simulink model "sia003A"  (R2023b)
settings: Solver=VariableStepAuto  StartTime=0.0  StopTime=10  FixedStep=0.001  RelTol=1e-3  EnableMultiTasking=on
values from neighbouring files (symbols this model uses):
  a1 = 0.040    (= 0.04)    [run_feedforward_experiment.m]
  a2 = 0.275    [run_feedforward_experiment.m]
  a3 = 0.025    [run_feedforward_experiment.m]
  d4 = 0.280    (= 0.28)    [run_feedforward_experiment.m]
  m = [0.167, 1, 0.5, 0.333, 0.25, 0.2]    [run_feedforward_experiment.m]
undefined symbols (not defined in the file or in its folder): d1, fc1, fc2, fc3, fc4, fc5, fc6, fv1, fv2, fv3, fv4, fv5, fv6, Ia1, Ia2, Ia3, Ia4, Ia5, Ia6, Ic111, Ic112, Ic113, Ic122, Ic123, Ic133, Ic211, Ic212, Ic213, Ic222, Ic223, Ic233, Ic311, Ic312, Ic313, Ic322, Ic323, Ic333, Ic411, Ic412, Ic413, Ic422, Ic423, Ic433, Ic511, Ic512, Ic513, Ic522, Ic523, Ic533, Ic611, Ic612, Ic613, Ic622, Ic623, Ic633, m1, m2, m3, m4, m5 ... (+22)
libraries: sm_lib x56, nesl_utility x31, slpidlib x12, simulink x8
(part 3 of 3)

== matlab function sia003A/Robot/Robot/robot/friction ==
  data: u input; y output; fv input; fc input
function y = fcn(u,fv,fc)
%#codegen


% fv1=100; fc1=80; fv2=150; fc2=100; fv3=100; fc3=50; fv4=80; fc4=80; fv5=50; fc5=30; fv6=30; fc6=10;
fv1=fv(1); fc1=fc(1); fv2=fv(2); fc2=fc(2); fv3=fv(3); fc3=fc(3); fv4=fv(4); fc4=fc(4); fv5=fv(5); fc5=fc(5); fv6=fv(6); fc6=fc(6);
y=[0;0;0;0;0;0];
y(1)=(fv1*u(1)+fc1*sign(u(1)));
y(2)=(fv2*u(2)+fc2*sign(u(2)));
y(3)=(fv3*u(3)+fc3*sign(u(3)));
y(4)=(fv4*u(4)+fc4*sign(u(4)));
y(5)=(fv5*u(5)+fc5*sign(u(5)));
y(6)=(fv6*u(6)+fc6*sign(u(6)));

end

== matlab function sia003A/Robot/Robot/robot/Jm ==
  data: u input; y output; Jm input
function y = fcn(u,Jm)
%#codegen

% Jm=[200; 250; 150; 100; 50; 20];%关节惯性
y = Jm.*u;
end

== matlab function sia003A/周期信号发生器 ==
  data: Amplitude parameter; Bias parameter; Frequency parameter; Phase parameter; out output; t_in input
function out=PeriodicSignallGenerator(Amplitude,Bias,Frequency, Phase,t_in)

    [m,n]=size(Amplitude);
    Amplitude=reshape(Amplitude,m*n,1);
    Bias=reshape(Bias,m*n,1);
    Frequency=reshape(Frequency,m*n,1);
    Phase=reshape(Phase,m*n,1);
    %规划
	ss=zeros(m*n,1);
	se=Amplitude;
	vs=zeros(m*n,1);
	ve=zeros(m*n,1);
	as=zeros(m*n,1);
	ae=zeros(m*n,1);
	js=zeros(m*n,1);
	je=zeros(m*n,1);
	tend=0.25./Frequency;

	tf=tend;
	tf2=tend.*tend;
	tf3=tend.*tend.*tend;
	tf4=tend.*tend.*tend.*tend;
	tf5=tend.*tend.*tend.*tend.*tend;
	tf6=tend.*tend.*tend.*tend.*tend.*tend;
	tf7=tend.*tend.*tend.*tend.*tend.*tend.*tend;

	b1=se-js./6.0.*tf3 - as./2.0.*tf2 - vs.*tf - ss;
	b2=ve-js./2.0.*tf2 - as.*tf - vs;
	b3=ae-js.*tf - as;
	b4=je-js;

    a=zeros(m*n,8);
	a(:,1)=ss;
	a(:,2)=vs;
	a(:,3)=as./2.0;
	a(:,4)=js./6.0;
	a(:,5)=(35.*b1)./tf4 - (15.*b2)./tf3 + (5.*b3)./(2.*tf2) - b4./(6.*tf);
	a(:,6)=(39.*b2)./tf4 - (84.*b1)./tf5 - (7.*b3)./tf3 + b4./(2.*tf2);
	a(:,7)=(70.*b1)./tf6 - (34.*b2)./tf5 + (13.*b3)./(2.*tf4) - b4./(2.*tf3);
	a(:,8)=(10.*b2)./tf6 - (20.*b1)./tf7 - (2.*b3)./tf5 + b4./(6.*tf4);
    
    %
    t_=zeros(m*n,1);
    t=zeros(m*n,1);
    ts=1.0./Frequency;
	t14=ts./4.0;
	t24=ts./2.0;
	t34=3.*ts./4.0;
	t44=ts;
	
    sign_=ones(m*n,1);
    %   
    for k=1:m*n
        t(k)=t_in+Phase(k);
        if (t(k)<0)
            sign_(k)=-1;
            t(k)=-t(k);
        end
        t(k)=t(k)-floor(t(k)/ts(k))*ts(k);
        if ((t(k)>=0)&&(t(k)<t14(k)))
            t_(k)=t(k);
        end
        if ((t(k)>=t14(k))&&(t(k)<t24(k)))
             t_(k)=t24(k)-t(k); 
        end
        if((t(k)>=t24(k))&&(t(k)<t34(k)))
             t_(k)=t(k)-t24(k);
             sign_(k)=-1.*sign_(k);
        end
        if((t(k)>=t34(k)))
             t_(k)=t44(k)-t(k);
             sign_(k)=-1.*sign_(k);        
        end
    

        if (t(k)>tend(k))
            t(k)=tend(k);
        end
        if (t(k)<0)
            t(k)=0;
        end
    end

    
	t2=t_.*t_;
	t3=t_.*t_.*t_;
	t4=t_.*t_.*t_.*t_;
	t5=t_.*t_.*t_.*t_.*t_;
	t6=t_.*t_.*t_.*t_.*t_.*t_;
	t7=t_.*t_.*t_.*t_.*t_.*t_.*t_;

	out =a(:,8).*t7 + a(:,7).*t6 + a(:,6).*t5 + a(:,5).*t4 + a(:,4).*t3 + a(:,3).*t2 + a(:,2).*t + a(:,1);
	out=sign_.*out+Bias;

end

== matlab function sia003A/dynamics + PID Control/Idynamics/Robot Dynamics ==
  data: q input; T output; qd input; qdd input

function T   = Idynamics( q,qd,qdd )
offset2=-pi/2;

s1=sin(q(1)); c1=cos(q(1)); 
s2=sin(q(2)+offset2); c2=cos(q(2)+offset2);
s3=sin(q(3)); c3=cos(q(3));
s4=sin(q(4)); c4=cos(q(4));
s5=sin(q(5)); c5=cos(q(5));
s6=sin(q(6)); c6=cos(q(6));

Q11=qd(1);  Q21=qd(2);  Q31=qd(3);  Q41=qd(4);  Q51=qd(5);  Q61=qd(6); 
Q12=qdd(1);  Q22=qdd(2);  Q32=qdd(3);  Q42=qdd(4);  Q52=qdd(5);  Q62=qdd(6);
f71=0;  f72=0;  f73=0;  n71=0;  n72=0;  n73=0;

%---------------------------------设置参数--------------------------------

% m1=0.00100000000000000;  m2=0.00100000000000000;  m3=0.00100000000000000;  m4=0.00100000000000000;  m5=0.00100000000000000;  m6=0.00100000000000000;
% 
% mc11=0;  mc12=0;  mc13=0;
% mc21=4651.50225394466;  mc22=-131.825587047461;  mc23=0;
% mc31=-60.5441532996453;  mc32=674.258060919694;  mc33=0;
% mc41=18.7559635838501;  mc42=-8.94631572009627;  mc43=0;
% mc51=39.1850949869383;  mc52=70.3651817994520;  mc53=0;
% mc61=-9.46764788612443;  mc62=-36.4261551831934;  mc63=0;%质心位置
% 
% 
% Ic111=0;  Ic122=0;  Ic133=2580.391811604250;  Ic112=0;  Ic113=0;  Ic123=0;
% Ic211=-2308.54980136788;  Ic222=-21636.4732184523;  Ic233=-19427.4931578430;  Ic212=-655.299381991673;  Ic213=-402.481626864736;  Ic223=1625.61432421119;
% Ic311=177.446872113322;  Ic322=-3.66559449877095;  Ic333=1225.66014585809;  Ic312=1065.32242628535;  Ic313=135.253022811379;  Ic323=-212.654795897439;
% Ic411=-856.449748636182;  Ic422=-0.351786169958710;  Ic433=637.546049655485;  Ic412=17.6321938869444;  Ic413=432.315615848409;  Ic423=528.159872075546;
% Ic511=53.5070403383571;  Ic522=-1.53547166913538;  Ic533=-275.931221064706;  Ic512=43.6352272669739;  Ic513=-110.142321946823;  Ic523=-292.481991287130;
% Ic611=89.4468595890859;  Ic622=-0.0896363564956364;  Ic633=183.333947383574;  Ic612=-31.1239742083191;  Ic613=40.1733539538204;  Ic623=-0.510715170309807;%惯性矩
% 
% g=9802.00;
% 
% %XB4
% % d1=342;a1=40;a2=275;a3=25;d4=280;dt=73;
% %XB6
% % d1=380;a1=30;a2=340;a3=35;d4=345;dt=90;
% %XB7
% d1=380;a1=30;a2=340;a3=35;d4=345;dt=87;
% 
% Ia1=0; Ia2=0; Ia3=-381.979781193985; Ia4=-848.046494253400; Ia5=106.880560008008; Ia6=-553.016107704353;%关节惯性
% fv1=14300.3219938765; fc1=10364.8985579369; fv2=77554.0985985479; fc2=17597.4704449446; fv3=13127.7878719491; fc3=8947.89951285878; 
% fv4=3252.91588327327; fc4=4394.56545040839; fv5=5533.12349479137; fc5=2614.97320533832; fv6=2209.46946763177; fc6=4156.29047300509;%粘滞摩擦,库伦摩擦

% m1=1.00000000000000;  m2=1.00000000000000;  m3=1.00000000000000;  m4=1.00000000000000;  m5=1.00000000000000;  m6=1.00000000000000;
% 
% mc11=0;  mc12=0;  mc13=0;
% mc21=4.65150225394466;  mc22=-0.131825587047461;  mc23=0;
% mc31=-0.0605441532996453;  mc32=0.674258060919694;  mc33=0;
% mc41=0.0187559635838501;  mc42=-0.00894631572009627;  mc43=0;
% mc51=0.0391850949869383;  mc52=0.0703651817994520;  mc53=0;
% mc61=-0.00946764788612443;  mc62=-0.0364261551831934;  mc63=0;%质心位置
% 
% Ic111=0;  Ic122=0;  Ic133=2.580391811604250;  Ic112=0;  Ic113=0;  Ic123=0;
% Ic211=-2.30854980136788;  Ic222=-21.6364732184523;  Ic233=-19.4274931578430;  Ic212=-0.655299381991673;  Ic213=-0.402481626864736;  Ic223=1.62561432421119;
% Ic311=0.177446872113322;  Ic322=-0.00366559449877095;  Ic333=1.22566014585809;  Ic312=1.06532242628535;  Ic313=0.135253022811379;  Ic323=-0.212654795897439;
% Ic411=-0.856449748636182;  Ic422=-0.000351786169958710;  Ic433=0.637546049655485;  Ic412=0.0176321938869444;  Ic413=0.432315615848409;  Ic423=0.528159872075546;
% Ic511=0.0535070403383571;  Ic522=-0.00153547166913538;  Ic533=-0.275931221064706;  Ic512=0.0436352272669739;  Ic513=-0.110142321946823;  Ic523=-0.292481991287130;
% Ic611=0.0894468595890859;  Ic622=-0.0000896363564956364;  Ic633=0.183333947383574;  Ic612=-0.0311239742083191;  Ic613=0.0401733539538204;  Ic623=-0.000510715170309807;%惯性矩
% 
% g=9.80200;
% 
% %XB4
% % d1=342;a1=40;a2=275;a3=25;d4=280;dt=73;
% %XB6
% % d1=380;a1=30;a2=340;a3=35;d4=345;dt=90;
% %XB7
% d1=0.380;a1=0.030;a2=0.340;a3=0.035;d4=0.345;dt=0.087;
% 
% Ia1=0; Ia2=0; Ia3=-0.381979781193985; Ia4=-0.848046494253400; Ia5=0.106880560008008; Ia6=-0.553016107704353;%关节惯性
% fv1=14.3003219938765; fc1=10.3648985579369; fv2=77.5540985985479; fc2=17.5974704449446; fv3=13.1277878719491; fc3=8.94789951285878; 
% fv4=3.25291588327327; fc4=4.39456545040839; fv5=5.53312349479137; fc5=2.61497320533832; fv6=2.20946946763177; fc6=4.15629047300509;%粘滞摩擦,库伦摩擦
% 
% % Ia1=0; Ia2=0; Ia3=0; Ia4=0; Ia5=0; Ia6=0;%关节惯性
% % fv1=0; fc1=0; fv2=0; fc2=0; fv3=0; fc3=0; 
% % fv4=0; fc4=0; fv5=0; fc5=0; fv6=0; fc6=0;%粘滞摩擦,库伦摩擦

m1=0.167;  m2=1;  m3=0.5;  m4=0.333;  m5=0.25;  m6=0.2;

mc11=0;  mc12=0;  mc13=0.2;
mc21=0.1291;  mc22=0;  mc23=3.3117;
mc31=1.6484;  mc32=0;  mc33=0.8748;
mc41=0.3200;  mc42=0.2324;  mc43=0.7083;
mc51=0.4574;  mc52=0;  mc53=0.6427;
mc61=0.3200;  mc62=-0.0513;  mc63=0.6417;%质心位置

Ic111=0;  Ic122=0;  Ic133=1.3676;  Ic112=0;  Ic113=0;  Ic123=0;
Ic211=8.8194;  Ic222=6.0549;  Ic233=0.9569;  Ic212=0;  Ic213=0;  Ic223=0;
Ic311=0.0332;  Ic322=1.8442;  Ic333=1.0560;  Ic312=0;  Ic313=0;  Ic323=0;
Ic411=0.1448;  Ic422=0.0015;  Ic433=0.0822;  Ic412=0;  Ic413=0;  Ic423=0;
Ic511=0;  Ic522=0.0121;  Ic533=0.0299;  Ic512=0;  Ic513=0;  Ic523=0;
Ic611=0.0134;  Ic622=0;  Ic633=0.0051;  Ic612=0;  Ic613=0;  Ic623=0;%惯性矩

g=9.80200;

%XB4
d1=0.342;a1=0.040;a2=0.275;a3=0.025;d4=0.280;dt=0.073;
%XB6
% d1=380;a1=30;a2=340;a3=35;d4=345;dt=90;
%XB7
% d1=0.380;a1=0.030;a2=0.340;a3=0.035;d4=0.345;dt=0.087;

Ia1=0; Ia2=0; Ia3=0; Ia4=0; Ia5=0; Ia6=0;%关节惯性
fv1=0; fc1=0; fv2=0; fc2=0; fv3=0; fc3=0; 
fv4=0; fc4=0; fv5=0; fc5=0; fv6=0; fc6=0;%粘滞摩擦,库伦摩擦



R01=[c1 -s1 0;
    s1 c1 0;
    0 0 1];
R12=[c2 -s2 0;
    0 0 1;
    -s2 -c2 0];
R23=[c3 -s3 0;
    s3 c3 0;
    0 0 1];
R34=[c4 -s4 0;
    0 0 1;
    -s4 -c4 0];
R45=[c5 -s5 0;
    0 0 -1;
    s5 c5 0];
R56=[c6 -s6 0;
    0 0 1;
    -s6 -c6 0];
R06=R01*R12*R23*R34*R45*R56;
R10=R01';R21=R12';R32=R23';R43=R34';R54=R45';R65=R56';
%R67=eye(3);

QZ1=[0;0;Q11];QZ2=[0;0;Q21];QZ3=[0;0;Q31];QZ4=[0;0;Q41];QZ5=[0;0;Q51];QZ6=[0;0;Q61];
QZ11=[0;0;Q12];QZ21=[0;0;Q22];QZ31=[0;0;Q32];QZ41=[0;0;Q42];QZ51=[0;0;Q52];QZ61=[0;0;Q62];
P01=[0;0;d1];P12=[a1;0;0];P23=[a2;0;0];P34=[a3;d4;0];P45=[0;0;0];P56=[0;0;0];P67=[0;0;dt];%下一个坐标系原点在当前坐标系的位置
Pc1=[mc11;mc12;mc13];Pc2=[mc21;mc22;mc23];Pc3=[mc31;mc32;mc33];Pc4=[mc41;mc42;mc43];Pc5=[mc51;mc52;mc53];Pc6=[mc61;mc62;mc63];%质心位置
Ic1=[Ic111 Ic112 Ic113;Ic112 Ic122 Ic123;Ic113 Ic123 Ic133];Ic2=[Ic211 Ic212 Ic213;Ic212 Ic222 Ic223;Ic213 Ic223 Ic233];Ic3=[Ic311 Ic312 Ic313;Ic312 Ic322 Ic323;Ic313 Ic323 Ic333];Ic4=[Ic411 Ic412 Ic413;Ic412 Ic422 Ic423;Ic413 Ic423 Ic433];Ic5=[Ic511 Ic512 Ic513;Ic512 Ic522 Ic523;Ic513 Ic523 Ic533];Ic6=[Ic611 Ic612 Ic613;Ic612 Ic622 Ic623;Ic613 Ic623 Ic633];%参考坐标在质心的惯性张量
f7=[f71;f72;f73];n7=[n71;n72;n73];


w0=[0;0;0];%基座角速度
w01=[0;0;0];%基座角加速度
v01=[0;0;g];%考虑重力影响

%速度、加速度向外递推
w1=R10*w0+QZ1;
w11=R10*w01+cross(R10*w0,QZ1)+QZ11;
v11=R10*(cross(w01,P01)+cross(w0,cross(w0,P01))+v01);
vc11=cross(w11,Pc1)+cross(w1,cross(w1,Pc1))+v11;
F1=m1*vc11;
N1=Ic1*w11+cross(w1,Ic1*w1);

w2=R21*w1+QZ2;
w21=R21*w11+cross(R21*w1,QZ2)+QZ21;
v21=R21*(cross(w11,P12)+cross(w1,cross(w1,P12))+v11);
vc21=cross(w21,Pc2)+cross(w2,cross(w2,Pc2))+v21;
F2=m2*vc21;
N2=Ic2*w21+cross(w2,Ic2*w2);

w3=R32*w2+QZ3;
w31=R32*w21+cross(R32*w2,QZ3)+QZ31;
v31=R32*(cross(w21,P23)+cross(w2,cross(w2,P23))+v21);
vc31=cross(w31,Pc3)+cross(w3,cross(w3,Pc3))+v31;
F3=m3*vc31;
N3=Ic3*w31+cross(w3,Ic3*w3);

w4=R43*w3+QZ4;
w41=R43*w31+cross(R43*w3,QZ4)+QZ41;
v41=R43*(cross(w31,P34)+cross(w3,cross(w3,P34))+v31);
vc41=cross(w41,Pc4)+cross(w4,cross(w4,Pc4))+v41;
F4=m4*vc41;
N4=Ic4*w41+cross(w4,Ic4*w4);

w5=R54*w4+QZ5;
w51=R54*w41+cross(R54*w4,QZ5)+QZ51;
v51=R54*(cross(w41,P45)+cross(w4,cross(w4,P45))+v41);
vc51=cross(w51,Pc5)+cross(w5,cross(w5,Pc5))+v51;
F5=m5*vc51;
N5=Ic5*w51+cross(w5,Ic5*w5);

w6=R65*w5+QZ6;
w61=R65*w51+cross(R65*w5,QZ6)+QZ61;
v61=R65*(cross(w51,P56)+cross(w5,cross(w5,P56))+v51);
vc61=cross(w61,Pc6)+cross(w6,cross(w6,Pc6))+v61;
F6=m6*vc61;
N6=Ic6*w61+cross(w6,Ic6*w6);

%力、力矩向内递推
f6=f7+F6;
n6=N6+n7+cross(Pc6,F6)+cross(P67,f7);
T6=n6'*[0;0;1];

f5=R56*f6+F5;
n5=N5+R56*n6+cross(Pc5,F5)+cross(P56,R56*f6);
T5=n5'*[0;0;1];

f4=R45*f5+F4;
n4=N4+R45*n5+cross(Pc4,F4)+cross(P45,R45*f5);
T4=n4'*[0;0;1];

f3=R34*f4+F3;
n3=N3+R34*n4+cross(Pc3,F3)+cross(P34,R34*f4);
T3=n3'*[0;0;1];

f2=R23*f3+F2;
n2=N2+R23*n3+cross(Pc2,F2)+cross(P23,R23*f3);
T2=n2'*[0;0;1];

f1=R12*f2+F1;
n1=N1+R12*n2+cross(Pc1,F1)+cross(P12,R12*f2);
T1=n1'*[0;0;1];

%加入关节惯性及摩擦模型
T1=T1+Ia1*Q12+fv1*Q11+fc1*sign(Q11);
T2=T2+Ia2*Q22+fv2*Q21+fc2*sign(Q21);
T3=T3+Ia3*Q32+fv3*Q31+fc3*sign(Q31);
T4=T4+Ia4*Q42+fv4*Q41+fc4*sign(Q41);
T5=T5+Ia5*Q52+fv5*Q51+fc5*sign(Q51);
T6=T6+Ia6*Q62+fv6*Q61+fc6*sign(Q61);
T=[T1;T2;T3;T4;T5;T6];

end
